simulink model "ALL_JP360_DBW_V6_5_1103"  (R2022a)
settings: Solver=FixedStepAuto  StartTime=0.0  StopTime=inf  FixedStep=0.01  RelTol=1e-3  EnableMultiTasking=on
model workspace (MAT data in the model file):
  g = 9.8
undefined symbols (not defined in the file or in its folder): canChannel, delta_v_p, IPM_Line_C0, IPM_Line_C1, IPM_Line_C2, IPM_Line_C3, M, M_p, MRR_ObjDistX, MRR_ObjDistY, MRR_ObjFusionCamID, MRR_ObjFusionSig, MRR_ObjID, MRR_ObjRelVelX, MRR_ObjRelVelY, MRR_ObjType, MRR_ObjUpdFlg, none, obj_vaild, untracktime, V, videoinput
libraries: canfdmsglib x230, canfdlib x76, slpidlib x24, simulink x18, dspstat3 x14, ctrlSharedLib x1, simulink_extras x1, imaqlib x1, realtime_pacer_lib x1, dspvision x1, visionsinks x1
(part 40 of 55)

== system ALL_JP360_DBW_V6_5_1103/MsgFromCAN/Subsystem/Subsystem3 ==
  VR_ADCU_MRR_ObjHeader_0x680FromOutData : Inport
  Bus Selector : BusSelector  OutputSignals=MRR_ObjDistX_07,MRR_ObjDistY_07,MRR_ObjExistProb_07,MRR_ObjFusionCamID_07,MRR_ObjFusionSig_07,MRR_ObjID_07,MRR_ObjMovingSts_07,MRR_ObjObstacleProb_07,MRR_ObjRelAccelX_07,MRR_ObjRelAccelY_07,MRR_ObjRelVelX_07,MRR_ObjRelVelY_07,MRR_ObjType_07,MRR_ObjUpdFlg_07
  Bus Selector1 : BusSelector  OutputSignals=MRR_ObjDistX_08,MRR_ObjDistY_08,MRR_ObjExistProb_08,MRR_ObjFusionCamID_08,MRR_ObjFusionSig_08,MRR_ObjID_08,MRR_ObjMovingSts_08,MRR_ObjObstacleProb_08,MRR_ObjRelAccelX_08,MRR_ObjRelAccelY_08,MRR_ObjRelVelX_08,MRR_ObjRelVelY_08,MRR_ObjType_08,MRR_ObjUpdFlg_08
  Data Type Conversion{,1..27} (28 alike) : DataTypeConversion  OutDataTypeStr=single  SaturateOnIntegerOverflow=off  RndMeth=Floor
  Mux : Mux  Inputs=14
  Mux1 : Mux  Inputs=14
  Out1 : Outport
  Out2 : Outport  Port=2
  wires:
  Data Type Conversion5/1 -> Mux/6
  Data Type Conversion3/1 -> Mux/4
  Data Type Conversion17/1 -> Mux1/3
  Data Type Conversion19/1 -> Mux1/5
  Data Type Conversion26/1 -> Mux1/12
  Data Type Conversion24/1 -> Mux1/10
  Data Type Conversion22/1 -> Mux1/8
  Data Type Conversion20/1 -> Mux1/6
  Data Type Conversion4/1 -> Mux/5
  Data Type Conversion2/1 -> Mux/3
  Data Type Conversion16/1 -> Mux1/2
  Data Type Conversion18/1 -> Mux1/4
  Data Type Conversion27/1 -> Mux1/13
  Data Type Conversion25/1 -> Mux1/11
  Data Type Conversion23/1 -> Mux1/9
  Data Type Conversion21/1 -> Mux1/7
  Data Type Conversion13/1 -> Mux/14
  Data Type Conversion11/1 -> Mux/12
  Data Type Conversion1/1 -> Mux/2
  Data Type Conversion15/1 -> Mux1/1
  Bus Selector1/11 -> Data Type Conversion25/1  "<MRR_ObjRelVelX_08>"
  Bus Selector1/13 -> Data Type Conversion27/1  "<MRR_ObjType_08>"
  Bus Selector1/10 -> Data Type Conversion24/1  "<MRR_ObjRelAccelY_08>"
  Bus Selector1/12 -> Data Type Conversion26/1  "<MRR_ObjRelVelY_08>"
  Bus Selector/3 -> Data Type Conversion2/1  "<MRR_ObjExistProb_07>"
  Bus Selector1/5 -> Data Type Conversion19/1  "<MRR_ObjFusionSig_08>"
  Bus Selector1/7 -> Data Type Conversion21/1  "<MRR_ObjMovingSts_08>"
  Bus Selector1/9 -> Data Type Conversion23/1  "<MRR_ObjRelAccelX_08>"
  Bus Selector/14 -> Data Type Conversion13/1  "<MRR_ObjUpdFlg_07>"
  Bus Selector1/4 -> Data Type Conversion18/1  "<MRR_ObjFusionCamID_08>"
  Bus Selector1/6 -> Data Type Conversion20/1  "<MRR_ObjID_08>"
  Bus Selector1/8 -> Data Type Conversion22/1  "<MRR_ObjObstacleProb_08>"
  Bus Selector1/3 -> Data Type Conversion17/1  "<MRR_ObjExistProb_08>"
  Bus Selector1/2 -> Data Type Conversion16/1  "<MRR_ObjDistY_08>"
  Bus Selector1/1 -> Data Type Conversion15/1  "<MRR_ObjDistX_08>"
  Data Type Conversion12/1 -> Mux/13
  Data Type Conversion10/1 -> Mux/11
  Data Type Conversion/1 -> Mux/1
  Data Type Conversion8/1 -> Mux/9
  Data Type Conversion6/1 -> Mux/7
  Data Type Conversion9/1 -> Mux/10
  Data Type Conversion7/1 -> Mux/8
  Bus Selector/1 -> Data Type Conversion/1  "<MRR_ObjDistX_07>"
  Mux/1 -> Out1/1
  Bus Selector/2 -> Data Type Conversion1/1  "<MRR_ObjDistY_07>"
  Bus Selector/4 -> Data Type Conversion3/1  "<MRR_ObjFusionCamID_07>"
  Bus Selector/5 -> Data Type Conversion4/1  "<MRR_ObjFusionSig_07>"
  Bus Selector/12 -> Data Type Conversion11/1  "<MRR_ObjRelVelY_07>"
  Bus Selector/10 -> Data Type Conversion9/1  "<MRR_ObjRelAccelY_07>"
  Bus Selector/8 -> Data Type Conversion7/1  "<MRR_ObjObstacleProb_07>"
  Bus Selector/6 -> Data Type Conversion5/1  "<MRR_ObjID_07>"
  Bus Selector/13 -> Data Type Conversion12/1  "<MRR_ObjType_07>"
  Bus Selector/11 -> Data Type Conversion10/1  "<MRR_ObjRelVelX_07>"
  Bus Selector/9 -> Data Type Conversion8/1  "<MRR_ObjRelAccelX_07>"
  Bus Selector/7 -> Data Type Conversion6/1  "<MRR_ObjMovingSts_07>"
  Mux1/1 -> Out2/1
  VR_ADCU_MRR_ObjHeader_0x680FromOutData/1 -> Bus Selector1/1, Bus Selector/1

== system ALL_JP360_DBW_V6_5_1103/MsgFromCAN/Subsystem/Subsystem4 ==
  VR_ADCU_MRR_ObjHeader_0x680FromOutData : Inport
  Bus Selector : BusSelector  OutputSignals=MRR_ObjDistX_09,MRR_ObjDistY_09,MRR_ObjExistProb_09,MRR_ObjFusionCamID_09,MRR_ObjFusionSig_09,MRR_ObjID_09,MRR_ObjMovingSts_09,MRR_ObjObstacleProb_09,MRR_ObjRelAccelX_09,MRR_ObjRelAccelY_09,MRR_ObjRelVelX_09,MRR_ObjRelVelY_09,MRR_ObjType_09,MRR_ObjUpdFlg_09
  Bus Selector1 : BusSelector  OutputSignals=MRR_ObjDistX_10,MRR_ObjDistY_10,MRR_ObjExistProb_10,MRR_ObjFusionCamID_10,MRR_ObjFusionSig_10,MRR_ObjID_10,MRR_ObjMovingSts_10,MRR_ObjObstacleProb_10,MRR_ObjRelAccelX_10,MRR_ObjRelAccelY_10,MRR_ObjRelVelX_10,MRR_ObjRelVelY_10,MRR_ObjType_10,MRR_ObjUpdFlg_10
  Data Type Conversion{,1..27} (28 alike) : DataTypeConversion  OutDataTypeStr=single  SaturateOnIntegerOverflow=off  RndMeth=Floor
  Mux : Mux  Inputs=14
  Mux1 : Mux  Inputs=14
  Out1 : Outport
  Out2 : Outport  Port=2
  wires:
  Mux/1 -> Out1/1
  Mux1/1 -> Out2/1
  VR_ADCU_MRR_ObjHeader_0x680FromOutData/1 -> Bus Selector/1, Bus Selector1/1
  Bus Selector/12 -> Data Type Conversion11/1  "<MRR_ObjRelVelY_09>"
  Bus Selector/11 -> Data Type Conversion10/1  "<MRR_ObjRelVelX_09>"
  Bus Selector/13 -> Data Type Conversion12/1  "<MRR_ObjType_09>"
  Bus Selector/10 -> Data Type Conversion9/1  "<MRR_ObjRelAccelY_09>"
  Bus Selector/14 -> Data Type Conversion13/1  "<MRR_ObjUpdFlg_09>"
  Bus Selector/9 -> Data Type Conversion8/1  "<MRR_ObjRelAccelX_09>"
  Bus Selector/8 -> Data Type Conversion7/1  "<MRR_ObjObstacleProb_09>"
  Bus Selector/7 -> Data Type Conversion6/1  "<MRR_ObjMovingSts_09>"
  Bus Selector/6 -> Data Type Conversion5/1  "<MRR_ObjID_09>"
  Bus Selector/5 -> Data Type Conversion4/1  "<MRR_ObjFusionSig_09>"
  Bus Selector/4 -> Data Type Conversion3/1  "<MRR_ObjFusionCamID_09>"
  Bus Selector/3 -> Data Type Conversion2/1  "<MRR_ObjExistProb_09>"
  Bus Selector/2 -> Data Type Conversion1/1  "<MRR_ObjDistY_09>"
  Bus Selector/1 -> Data Type Conversion/1  "<MRR_ObjDistX_09>"
  Data Type Conversion11/1 -> Mux/12
  Data Type Conversion10/1 -> Mux/11
  Data Type Conversion12/1 -> Mux/13
  Data Type Conversion9/1 -> Mux/10
  Data Type Conversion13/1 -> Mux/14
  Data Type Conversion8/1 -> Mux/9
  Data Type Conversion7/1 -> Mux/8
  Data Type Conversion6/1 -> Mux/7
  Data Type Conversion5/1 -> Mux/6
  Data Type Conversion4/1 -> Mux/5
  Data Type Conversion3/1 -> Mux/4
  Data Type Conversion2/1 -> Mux/3
  Data Type Conversion1/1 -> Mux/2
  Data Type Conversion/1 -> Mux/1
  Bus Selector1/1 -> Data Type Conversion14/1  "<MRR_ObjDistX_10>"
  Bus Selector1/2 -> Data Type Conversion15/1  "<MRR_ObjDistY_10>"
  Bus Selector1/3 -> Data Type Conversion16/1  "<MRR_ObjExistProb_10>"
  Bus Selector1/4 -> Data Type Conversion17/1  "<MRR_ObjFusionCamID_10>"
  Bus Selector1/5 -> Data Type Conversion18/1  "<MRR_ObjFusionSig_10>"
  Bus Selector1/6 -> Data Type Conversion19/1  "<MRR_ObjID_10>"
  Bus Selector1/7 -> Data Type Conversion20/1  "<MRR_ObjMovingSts_10>"
  Bus Selector1/8 -> Data Type Conversion21/1  "<MRR_ObjObstacleProb_10>"
  Bus Selector1/9 -> Data Type Conversion22/1  "<MRR_ObjRelAccelX_10>"
  Bus Selector1/10 -> Data Type Conversion23/1  "<MRR_ObjRelAccelY_10>"
  Bus Selector1/11 -> Data Type Conversion24/1  "<MRR_ObjRelVelX_10>"
  Bus Selector1/12 -> Data Type Conversion25/1  "<MRR_ObjRelVelY_10>"
  Bus Selector1/13 -> Data Type Conversion26/1  "<MRR_ObjType_10>"
  Bus Selector1/14 -> Data Type Conversion27/1  "<MRR_ObjUpdFlg_10>"
  Data Type Conversion14/1 -> Mux1/1
  Data Type Conversion15/1 -> Mux1/2
  Data Type Conversion16/1 -> Mux1/3
  Data Type Conversion17/1 -> Mux1/4
  Data Type Conversion18/1 -> Mux1/5
  Data Type Conversion19/1 -> Mux1/6
  Data Type Conversion20/1 -> Mux1/7
  Data Type Conversion21/1 -> Mux1/8
  Data Type Conversion22/1 -> Mux1/9
  Data Type Conversion23/1 -> Mux1/10
  Data Type Conversion24/1 -> Mux1/11
  Data Type Conversion25/1 -> Mux1/12
  Data Type Conversion26/1 -> Mux1/13
  Data Type Conversion27/1 -> Mux1/14

== system ALL_JP360_DBW_V6_5_1103/MsgFromCAN/Subsystem/Subsystem5 ==
  VR_ADCU_MRR_ObjHeader_0x680FromOutData : Inport
  Bus Selector : BusSelector  OutputSignals=MRR_ObjDistX_11,MRR_ObjDistY_11,MRR_ObjExistProb_11,MRR_ObjFusionCamID_11,MRR_ObjFusionSig_11,MRR_ObjID_11,MRR_ObjMovingSts_11,MRR_ObjObstacleProb_11,MRR_ObjRelAccelX_11,MRR_ObjRelAccelY_11,MRR_ObjRelVelX_11,MRR_ObjRelVelY_11,MRR_ObjType_11,MRR_ObjUpdFlg_11
  Bus Selector1 : BusSelector  OutputSignals=MRR_ObjDistX_12,MRR_ObjDistY_12,MRR_ObjExistProb_12,MRR_ObjFusionCamID_12,MRR_ObjFusionSig_12,MRR_ObjID_12,MRR_ObjMovingSts_12,MRR_ObjObstacleProb_12,MRR_ObjRelAccelX_12,MRR_ObjRelAccelY_12,MRR_ObjRelVelX_12,MRR_ObjRelVelY_12,MRR_ObjType_12,MRR_ObjUpdFlg_12
  Data Type Conversion{,1..27} (28 alike) : DataTypeConversion  OutDataTypeStr=single  SaturateOnIntegerOverflow=off  RndMeth=Floor
  Mux : Mux  Inputs=14
  Mux1 : Mux  Inputs=14
  Out1 : Outport
  Out2 : Outport  Port=2
  wires:
  VR_ADCU_MRR_ObjHeader_0x680FromOutData/1 -> Bus Selector1/1, Bus Selector/1
  Mux1/1 -> Out2/1
  Mux/1 -> Out1/1
  Bus Selector/10 -> Data Type Conversion9/1  "<MRR_ObjRelAccelY_11>"
  Bus Selector/11 -> Data Type Conversion10/1  "<MRR_ObjRelVelX_11>"
  Bus Selector/9 -> Data Type Conversion8/1  "<MRR_ObjRelAccelX_11>"
  Bus Selector/12 -> Data Type Conversion11/1  "<MRR_ObjRelVelY_11>"
  Bus Selector/8 -> Data Type Conversion7/1  "<MRR_ObjObstacleProb_11>"
  Bus Selector/13 -> Data Type Conversion12/1  "<MRR_ObjType_11>"
  Bus Selector/7 -> Data Type Conversion6/1  "<MRR_ObjMovingSts_11>"
  Bus Selector/14 -> Data Type Conversion13/1  "<MRR_ObjUpdFlg_11>"
  Bus Selector/6 -> Data Type Conversion5/1  "<MRR_ObjID_11>"
  Bus Selector/5 -> Data Type Conversion4/1  "<MRR_ObjFusionSig_11>"
  Bus Selector/4 -> Data Type Conversion3/1  "<MRR_ObjFusionCamID_11>"
  Bus Selector/3 -> Data Type Conversion2/1  "<MRR_ObjExistProb_11>"
  Bus Selector/2 -> Data Type Conversion1/1  "<MRR_ObjDistY_11>"
  Bus Selector/1 -> Data Type Conversion/1  "<MRR_ObjDistX_11>"
  Data Type Conversion9/1 -> Mux/10
  Data Type Conversion10/1 -> Mux/11
  Data Type Conversion8/1 -> Mux/9
  Data Type Conversion11/1 -> Mux/12
  Data Type Conversion7/1 -> Mux/8
  Data Type Conversion12/1 -> Mux/13
  Data Type Conversion6/1 -> Mux/7
  Data Type Conversion13/1 -> Mux/14
  Data Type Conversion5/1 -> Mux/6
  Data Type Conversion4/1 -> Mux/5
  Data Type Conversion3/1 -> Mux/4
  Data Type Conversion2/1 -> Mux/3
  Data Type Conversion1/1 -> Mux/2
  Data Type Conversion/1 -> Mux/1
  Bus Selector1/1 -> Data Type Conversion14/1  "<MRR_ObjDistX_12>"
  Bus Selector1/2 -> Data Type Conversion15/1  "<MRR_ObjDistY_12>"
  Bus Selector1/3 -> Data Type Conversion16/1  "<MRR_ObjExistProb_12>"
  Bus Selector1/4 -> Data Type Conversion17/1  "<MRR_ObjFusionCamID_12>"
  Bus Selector1/5 -> Data Type Conversion18/1  "<MRR_ObjFusionSig_12>"
  Bus Selector1/6 -> Data Type Conversion19/1  "<MRR_ObjID_12>"
  Bus Selector1/7 -> Data Type Conversion20/1  "<MRR_ObjMovingSts_12>"
  Bus Selector1/8 -> Data Type Conversion21/1  "<MRR_ObjObstacleProb_12>"
  Bus Selector1/9 -> Data Type Conversion22/1  "<MRR_ObjRelAccelX_12>"
  Bus Selector1/10 -> Data Type Conversion23/1  "<MRR_ObjRelAccelY_12>"
  Bus Selector1/11 -> Data Type Conversion24/1  "<MRR_ObjRelVelX_12>"
  Bus Selector1/12 -> Data Type Conversion25/1  "<MRR_ObjRelVelY_12>"
  Bus Selector1/13 -> Data Type Conversion26/1  "<MRR_ObjType_12>"
  Bus Selector1/14 -> Data Type Conversion27/1  "<MRR_ObjUpdFlg_12>"
  Data Type Conversion14/1 -> Mux1/1
  Data Type Conversion15/1 -> Mux1/2
  Data Type Conversion16/1 -> Mux1/3
  Data Type Conversion17/1 -> Mux1/4
  Data Type Conversion18/1 -> Mux1/5
  Data Type Conversion19/1 -> Mux1/6
  Data Type Conversion20/1 -> Mux1/7
  Data Type Conversion21/1 -> Mux1/8
  Data Type Conversion22/1 -> Mux1/9
  Data Type Conversion23/1 -> Mux1/10
  Data Type Conversion24/1 -> Mux1/11
  Data Type Conversion25/1 -> Mux1/12
  Data Type Conversion26/1 -> Mux1/13
  Data Type Conversion27/1 -> Mux1/14

== system ALL_JP360_DBW_V6_5_1103/MsgFromCAN/Subsystem/Subsystem6 ==
  VR_ADCU_MRR_ObjHeader_0x680FromOutData : Inport
  Bus Selector : BusSelector  OutputSignals=MRR_ObjDistX_13,MRR_ObjDistY_13,MRR_ObjExistProb_13,MRR_ObjFusionCamID_13,MRR_ObjFusionSig_13,MRR_ObjID_13,MRR_ObjMovingSts_13,MRR_ObjObstacleProb_13,MRR_ObjRelAccelX_13,MRR_ObjRelAccelY_13,MRR_ObjRelVelX_13,MRR_ObjRelVelY_13,MRR_ObjType_13,MRR_ObjUpdFlg_13
  Bus Selector1 : BusSelector  OutputSignals=MRR_ObjDistX_14,MRR_ObjDistY_14,MRR_ObjExistProb_14,MRR_ObjFusionCamID_14,MRR_ObjFusionSig_14,MRR_ObjID_14,MRR_ObjMovingSts_14,MRR_ObjObstacleProb_14,MRR_ObjRelAccelX_14,MRR_ObjRelAccelY_14,MRR_ObjRelVelX_14,MRR_ObjRelVelY_14,MRR_ObjType_14,MRR_ObjUpdFlg_14
  Data Type Conversion{,1..27} (28 alike) : DataTypeConversion  OutDataTypeStr=single  SaturateOnIntegerOverflow=off  RndMeth=Floor
  Mux : Mux  Inputs=14
  Mux1 : Mux  Inputs=14
  Out1 : Outport
  Out2 : Outport  Port=2
  wires:
  Bus Selector/13 -> Data Type Conversion12/1  "<MRR_ObjType_13>"
  Bus Selector/1 -> Data Type Conversion/1  "<MRR_ObjDistX_13>"
  Data Type Conversion4/1 -> Mux/5
  Bus Selector1/5 -> Data Type Conversion18/1  "<MRR_ObjFusionSig_14>"
  Bus Selector1/7 -> Data Type Conversion20/1  "<MRR_ObjMovingSts_14>"
  Data Type Conversion27/1 -> Mux1/14
  Data Type Conversion25/1 -> Mux1/12
  Data Type Conversion23/1 -> Mux1/10
  Bus Selector/14 -> Data Type Conversion13/1  "<MRR_ObjUpdFlg_13>"
  Bus Selector/12 -> Data Type Conversion11/1  "<MRR_ObjRelVelY_13>"
  Data Type Conversion5/1 -> Mux/6
  Data Type Conversion3/1 -> Mux/4
  Bus Selector1/4 -> Data Type Conversion17/1  "<MRR_ObjFusionCamID_14>"
  Bus Selector1/6 -> Data Type Conversion19/1  "<MRR_ObjID_14>"
  Data Type Conversion26/1 -> Mux1/13
  Data Type Conversion24/1 -> Mux1/11
  Bus Selector1/2 -> Data Type Conversion15/1  "<MRR_ObjDistY_14>"
  Data Type Conversion17/1 -> Mux1/4
  Data Type Conversion19/1 -> Mux1/6
  Data Type Conversion22/1 -> Mux1/9
  Data Type Conversion20/1 -> Mux1/7
  Bus Selector/2 -> Data Type Conversion1/1  "<MRR_ObjDistY_13>"
  Data Type Conversion2/1 -> Mux/3
  Data Type Conversion16/1 -> Mux1/3
  Data Type Conversion18/1 -> Mux1/5
  Data Type Conversion21/1 -> Mux1/8
  Data Type Conversion13/1 -> Mux/14
  Data Type Conversion11/1 -> Mux/12
  Data Type Conversion1/1 -> Mux/2
  Data Type Conversion15/1 -> Mux1/2
  Data Type Conversion12/1 -> Mux/13
  Data Type Conversion10/1 -> Mux/11
  Data Type Conversion/1 -> Mux/1
  Data Type Conversion14/1 -> Mux1/1
  Data Type Conversion8/1 -> Mux/9
  Data Type Conversion6/1 -> Mux/7
  Bus Selector1/8 -> Data Type Conversion21/1  "<MRR_ObjObstacleProb_14>"
  Bus Selector1/10 -> Data Type Conversion23/1  "<MRR_ObjRelAccelY_14>"
  Bus Selector1/12 -> Data Type Conversion25/1  "<MRR_ObjRelVelY_14>"
  Bus Selector1/14 -> Data Type Conversion27/1  "<MRR_ObjUpdFlg_14>"
  Data Type Conversion9/1 -> Mux/10
  Data Type Conversion7/1 -> Mux/8
  Bus Selector1/9 -> Data Type Conversion22/1  "<MRR_ObjRelAccelX_14>"
  Bus Selector1/11 -> Data Type Conversion24/1  "<MRR_ObjRelVelX_14>"
  Bus Selector1/13 -> Data Type Conversion26/1  "<MRR_ObjType_14>"
  Bus Selector1/3 -> Data Type Conversion16/1  "<MRR_ObjExistProb_14>"
  Bus Selector1/1 -> Data Type Conversion14/1  "<MRR_ObjDistX_14>"
  Bus Selector/3 -> Data Type Conversion2/1  "<MRR_ObjExistProb_13>"
  Bus Selector/10 -> Data Type Conversion9/1  "<MRR_ObjRelAccelY_13>"
  Bus Selector/8 -> Data Type Conversion7/1  "<MRR_ObjObstacleProb_13>"
  Bus Selector/6 -> Data Type Conversion5/1  "<MRR_ObjID_13>"
  Bus Selector/4 -> Data Type Conversion3/1  "<MRR_ObjFusionCamID_13>"
  Bus Selector/11 -> Data Type Conversion10/1  "<MRR_ObjRelVelX_13>"
  Bus Selector/9 -> Data Type Conversion8/1  "<MRR_ObjRelAccelX_13>"
  Bus Selector/7 -> Data Type Conversion6/1  "<MRR_ObjMovingSts_13>"
  Bus Selector/5 -> Data Type Conversion4/1  "<MRR_ObjFusionSig_13>"
  Mux/1 -> Out1/1
  Mux1/1 -> Out2/1
  VR_ADCU_MRR_ObjHeader_0x680FromOutData/1 -> Bus Selector/1, Bus Selector1/1

== system ALL_JP360_DBW_V6_5_1103/MsgFromCAN/Subsystem/Subsystem7 ==
  VR_ADCU_MRR_ObjHeader_0x680FromOutData : Inport
  Bus Selector : BusSelector  OutputSignals=MRR_ObjDistX_15,MRR_ObjDistY_15,MRR_ObjExistProb_15,MRR_ObjFusionCamID_15,MRR_ObjFusionSig_15,MRR_ObjID_15,MRR_ObjMovingSts_15,MRR_ObjObstacleProb_15,MRR_ObjRelAccelX_15,MRR_ObjRelAccelY_15,MRR_ObjRelVelX_15,MRR_ObjRelVelY_15,MRR_ObjType_15,MRR_ObjUpdFlg_15
  Bus Selector1 : BusSelector  OutputSignals=MRR_ObjDistX_16,MRR_ObjDistY_16,MRR_ObjExistProb_16,MRR_ObjFusionCamID_16,MRR_ObjFusionSig_16,MRR_ObjID_16,MRR_ObjMovingSts_16,MRR_ObjObstacleProb_16,MRR_ObjRelAccelX_16,MRR_ObjRelAccelY_16,MRR_ObjRelVelX_16,MRR_ObjRelVelY_16,MRR_ObjType_16,MRR_ObjUpdFlg_16
  Data Type Conversion{,1..27} (28 alike) : DataTypeConversion  OutDataTypeStr=single  SaturateOnIntegerOverflow=off  RndMeth=Floor
  Mux : Mux  Inputs=14
  Mux1 : Mux  Inputs=14
  Out1 : Outport
  Out2 : Outport  Port=2
  wires:
  Bus Selector1/12 -> Data Type Conversion27/1  "<MRR_ObjRelVelY_16>"
  Bus Selector1/10 -> Data Type Conversion25/1  "<MRR_ObjRelAccelY_16>"
  Bus Selector1/11 -> Data Type Conversion26/1  "<MRR_ObjRelVelX_16>"
  Bus Selector1/9 -> Data Type Conversion24/1  "<MRR_ObjRelAccelX_16>"
  Bus Selector1/7 -> Data Type Conversion22/1  "<MRR_ObjMovingSts_16>"
  Bus Selector1/5 -> Data Type Conversion20/1  "<MRR_ObjFusionSig_16>"
  Bus Selector/14 -> Data Type Conversion13/1  "<MRR_ObjUpdFlg_15>"
  Bus Selector1/4 -> Data Type Conversion19/1  "<MRR_ObjFusionCamID_16>"
  Bus Selector1/8 -> Data Type Conversion23/1  "<MRR_ObjObstacleProb_16>"
  Bus Selector1/6 -> Data Type Conversion21/1  "<MRR_ObjID_16>"
  Bus Selector1/3 -> Data Type Conversion18/1  "<MRR_ObjExistProb_16>"
  Mux1/1 -> Out2/1
  Bus Selector/1 -> Data Type Conversion/1  "<MRR_ObjDistX_15>"
  Bus Selector1/2 -> Data Type Conversion17/1  "<MRR_ObjDistY_16>"
  VR_ADCU_MRR_ObjHeader_0x680FromOutData/1 -> Bus Selector/1, Bus Selector1/1
  Bus Selector1/1 -> Data Type Conversion16/1  "<MRR_ObjDistX_16>"
  Data Type Conversion8/1 -> Mux/9
  Data Type Conversion6/1 -> Mux/7
  Data Type Conversion4/1 -> Mux/5
  Data Type Conversion27/1 -> Mux1/12
  Data Type Conversion7/1 -> Mux/8
  Data Type Conversion5/1 -> Mux/6
  Data Type Conversion3/1 -> Mux/4
  Data Type Conversion26/1 -> Mux1/11
  Data Type Conversion2/1 -> Mux/3
  Data Type Conversion21/1 -> Mux1/6
  Data Type Conversion23/1 -> Mux1/8
  Data Type Conversion25/1 -> Mux1/10
  Bus Selector/2 -> Data Type Conversion1/1  "<MRR_ObjDistY_15>"
  Data Type Conversion19/1 -> Mux1/4
  Data Type Conversion20/1 -> Mux1/5
  Data Type Conversion22/1 -> Mux1/7
  Data Type Conversion24/1 -> Mux1/9
  Data Type Conversion12/1 -> Mux/13
  Data Type Conversion16/1 -> Mux1/1
  Data Type Conversion18/1 -> Mux1/3
  Data Type Conversion13/1 -> Mux/14
  Data Type Conversion11/1 -> Mux/12
  Data Type Conversion17/1 -> Mux1/2
  Data Type Conversion10/1 -> Mux/11
  Data Type Conversion/1 -> Mux/1
  Data Type Conversion1/1 -> Mux/2
  Mux/1 -> Out1/1
  Data Type Conversion9/1 -> Mux/10
  Bus Selector/3 -> Data Type Conversion2/1  "<MRR_ObjExistProb_15>"
  Bus Selector/4 -> Data Type Conversion3/1  "<MRR_ObjFusionCamID_15>"
  Bus Selector/5 -> Data Type Conversion4/1  "<MRR_ObjFusionSig_15>"
  Bus Selector/12 -> Data Type Conversion11/1  "<MRR_ObjRelVelY_15>"
  Bus Selector/10 -> Data Type Conversion9/1  "<MRR_ObjRelAccelY_15>"
  Bus Selector/8 -> Data Type Conversion7/1  "<MRR_ObjObstacleProb_15>"
  Bus Selector/6 -> Data Type Conversion5/1  "<MRR_ObjID_15>"
  Bus Selector/13 -> Data Type Conversion12/1  "<MRR_ObjType_15>"
  Bus Selector/11 -> Data Type Conversion10/1  "<MRR_ObjRelVelX_15>"
  Bus Selector/9 -> Data Type Conversion8/1  "<MRR_ObjRelAccelX_15>"
  Bus Selector/7 -> Data Type Conversion6/1  "<MRR_ObjMovingSts_15>"

== system ALL_JP360_DBW_V6_5_1103/MsgFromCAN/Subsystem/Subsystem8 ==
  VR_ADCU_MRR_ObjHeader_0x680FromOutData : Inport
  Bus Selector : BusSelector  OutputSignals=MRR_ObjDistX_17,MRR_ObjDistY_17,MRR_ObjExistProb_17,MRR_ObjFusionCamID_17,MRR_ObjFusionSig_17,MRR_ObjID_17,MRR_ObjMovingSts_17,MRR_ObjObstacleProb_17,MRR_ObjRelAccelX_17,MRR_ObjRelAccelY_17,MRR_ObjRelVelX_17,MRR_ObjRelVelY_17,MRR_ObjType_17,MRR_ObjUpdFlg_17
  Bus Selector1 : BusSelector  OutputSignals=MRR_ObjDistX_18,MRR_ObjDistY_18,MRR_ObjExistProb_18,MRR_ObjFusionCamID_18,MRR_ObjFusionSig_18,MRR_ObjID_18,MRR_ObjMovingSts_18,MRR_ObjObstacleProb_18,MRR_ObjRelAccelX_18,MRR_ObjRelAccelY_18,MRR_ObjRelVelX_18,MRR_ObjRelVelY_18,MRR_ObjType_18,MRR_ObjUpdFlg_18
  Data Type Conversion{,1..27} (28 alike) : DataTypeConversion  OutDataTypeStr=single  SaturateOnIntegerOverflow=off  RndMeth=Floor
  Mux : Mux  Inputs=14
  Mux1 : Mux  Inputs=14
  Out1 : Outport
  Out2 : Outport  Port=2
  wires:
  Data Type Conversion4/1 -> Mux/5
  Data Type Conversion6/1 -> Mux/7
  Data Type Conversion27/1 -> Mux1/14
  Data Type Conversion25/1 -> Mux1/12
  Data Type Conversion3/1 -> Mux/4
  Data Type Conversion5/1 -> Mux/6
  Data Type Conversion7/1 -> Mux/8
  Data Type Conversion26/1 -> Mux1/13
  Data Type Conversion19/1 -> Mux1/6
  Data Type Conversion24/1 -> Mux1/11
  Data Type Conversion22/1 -> Mux1/9
  Data Type Conversion20/1 -> Mux1/7
  Data Type Conversion2/1 -> Mux/3
  Data Type Conversion18/1 -> Mux1/5
  Data Type Conversion23/1 -> Mux1/10
  Data Type Conversion21/1 -> Mux1/8
  Data Type Conversion11/1 -> Mux/12
  Data Type Conversion13/1 -> Mux/14
  Data Type Conversion15/1 -> Mux1/2
  Data Type Conversion17/1 -> Mux1/4
  Data Type Conversion10/1 -> Mux/11
  Data Type Conversion12/1 -> Mux/13
  Data Type Conversion14/1 -> Mux1/1
  Data Type Conversion16/1 -> Mux1/3
  Bus Selector1/12 -> Data Type Conversion25/1  "<MRR_ObjRelVelY_18>"
  Bus Selector1/14 -> Data Type Conversion27/1  "<MRR_ObjUpdFlg_18>"
  Bus Selector1/13 -> Data Type Conversion26/1  "<MRR_ObjType_18>"
  Mux1/1 -> Out2/1
  Bus Selector1/5 -> Data Type Conversion18/1  "<MRR_ObjFusionSig_18>"
  Bus Selector1/7 -> Data Type Conversion20/1  "<MRR_ObjMovingSts_18>"
  Bus Selector1/9 -> Data Type Conversion22/1  "<MRR_ObjRelAccelX_18>"
  Bus Selector1/11 -> Data Type Conversion24/1  "<MRR_ObjRelVelX_18>"
  Bus Selector1/4 -> Data Type Conversion17/1  "<MRR_ObjFusionCamID_18>"
  Bus Selector1/6 -> Data Type Conversion19/1  "<MRR_ObjID_18>"
  Bus Selector1/8 -> Data Type Conversion21/1  "<MRR_ObjObstacleProb_18>"
  Bus Selector1/10 -> Data Type Conversion23/1  "<MRR_ObjRelAccelY_18>"
  Bus Selector1/3 -> Data Type Conversion16/1  "<MRR_ObjExistProb_18>"
  Data Type Conversion1/1 -> Mux/2
  Bus Selector1/2 -> Data Type Conversion15/1  "<MRR_ObjDistY_18>"
  Data Type Conversion8/1 -> Mux/9
  Bus Selector1/1 -> Data Type Conversion14/1  "<MRR_ObjDistX_18>"
  Data Type Conversion9/1 -> Mux/10
  Data Type Conversion/1 -> Mux/1
  Bus Selector/8 -> Data Type Conversion7/1  "<MRR_ObjObstacleProb_17>"
  Bus Selector/10 -> Data Type Conversion9/1  "<MRR_ObjRelAccelY_17>"
  Bus Selector/12 -> Data Type Conversion11/1  "<MRR_ObjRelVelY_17>"
  Bus Selector/14 -> Data Type Conversion13/1  "<MRR_ObjUpdFlg_17>"
  Bus Selector/3 -> Data Type Conversion2/1  "<MRR_ObjExistProb_17>"
  Bus Selector/9 -> Data Type Conversion8/1  "<MRR_ObjRelAccelX_17>"
  Bus Selector/11 -> Data Type Conversion10/1  "<MRR_ObjRelVelX_17>"
  Bus Selector/13 -> Data Type Conversion12/1  "<MRR_ObjType_17>"
  Bus Selector/5 -> Data Type Conversion4/1  "<MRR_ObjFusionSig_17>"
  Bus Selector/7 -> Data Type Conversion6/1  "<MRR_ObjMovingSts_17>"
  Bus Selector/4 -> Data Type Conversion3/1  "<MRR_ObjFusionCamID_17>"
  Bus Selector/6 -> Data Type Conversion5/1  "<MRR_ObjID_17>"
  Bus Selector/1 -> Data Type Conversion/1  "<MRR_ObjDistX_17>"
  Bus Selector/2 -> Data Type Conversion1/1  "<MRR_ObjDistY_17>"
  Mux/1 -> Out1/1
  VR_ADCU_MRR_ObjHeader_0x680FromOutData/1 -> Bus Selector/1, Bus Selector1/1

== system ALL_JP360_DBW_V6_5_1103/MsgFromCAN/Subsystem/Subsystem9 ==
  VR_ADCU_MRR_ObjHeader_0x680FromOutData : Inport
  Bus Selector : BusSelector  OutputSignals=MRR_ObjDistX_19,MRR_ObjDistY_19,MRR_ObjExistProb_19,MRR_ObjFusionCamID_19,MRR_ObjFusionSig_19,MRR_ObjID_19,MRR_ObjMovingSts_19,MRR_ObjObstacleProb_19,MRR_ObjRelAccelX_19,MRR_ObjRelAccelY_19,MRR_ObjRelVelX_19,MRR_ObjRelVelY_19,MRR_ObjType_19,MRR_ObjUpdFlg_19
  Bus Selector1 : BusSelector  OutputSignals=MRR_ObjDistX_20,MRR_ObjDistY_20,MRR_ObjExistProb_20,MRR_ObjFusionCamID_20,MRR_ObjFusionSig_20,MRR_ObjID_20,MRR_ObjMovingSts_20,MRR_ObjObstacleProb_20,MRR_ObjRelAccelX_20,MRR_ObjRelAccelY_20,MRR_ObjRelVelX_20,MRR_ObjRelVelY_20,MRR_ObjType_20,MRR_ObjUpdFlg_20
  Data Type Conversion{,1..27} (28 alike) : DataTypeConversion  OutDataTypeStr=single  SaturateOnIntegerOverflow=off  RndMeth=Floor
  Mux : Mux  Inputs=14
  Mux1 : Mux  Inputs=14
  Out1 : Outport
  Out2 : Outport  Port=2
  wires:
  VR_ADCU_MRR_ObjHeader_0x680FromOutData/1 -> Bus Selector1/1, Bus Selector/1
  Mux1/1 -> Out2/1
  Mux/1 -> Out1/1
  Bus Selector/11 -> Data Type Conversion10/1  "<MRR_ObjRelVelX_19>"
  Bus Selector/12 -> Data Type Conversion11/1  "<MRR_ObjRelVelY_19>"
  Bus Selector/10 -> Data Type Conversion9/1  "<MRR_ObjRelAccelY_19>"
  Bus Selector/13 -> Data Type Conversion12/1  "<MRR_ObjType_19>"
  Bus Selector/9 -> Data Type Conversion8/1  "<MRR_ObjRelAccelX_19>"
  Bus Selector/14 -> Data Type Conversion13/1  "<MRR_ObjUpdFlg_19>"
  Bus Selector/8 -> Data Type Conversion7/1  "<MRR_ObjObstacleProb_19>"
  Bus Selector/7 -> Data Type Conversion6/1  "<MRR_ObjMovingSts_19>"
  Bus Selector/6 -> Data Type Conversion5/1  "<MRR_ObjID_19>"
  Bus Selector/5 -> Data Type Conversion4/1  "<MRR_ObjFusionSig_19>"
  Bus Selector/4 -> Data Type Conversion3/1  "<MRR_ObjFusionCamID_19>"
  Bus Selector/3 -> Data Type Conversion2/1  "<MRR_ObjExistProb_19>"
  Bus Selector/2 -> Data Type Conversion1/1  "<MRR_ObjDistY_19>"
  Bus Selector/1 -> Data Type Conversion/1  "<MRR_ObjDistX_19>"
  Data Type Conversion10/1 -> Mux/11
  Data Type Conversion11/1 -> Mux/12
  Data Type Conversion9/1 -> Mux/10
  Data Type Conversion12/1 -> Mux/13
  Data Type Conversion8/1 -> Mux/9
  Data Type Conversion13/1 -> Mux/14
  Data Type Conversion7/1 -> Mux/8
  Data Type Conversion6/1 -> Mux/7
  Data Type Conversion5/1 -> Mux/6
  Data Type Conversion4/1 -> Mux/5
  Data Type Conversion3/1 -> Mux/4
  Data Type Conversion2/1 -> Mux/3
  Data Type Conversion1/1 -> Mux/2
  Data Type Conversion/1 -> Mux/1
  Bus Selector1/1 -> Data Type Conversion14/1  "<MRR_ObjDistX_20>"
  Bus Selector1/2 -> Data Type Conversion15/1  "<MRR_ObjDistY_20>"
  Bus Selector1/3 -> Data Type Conversion16/1  "<MRR_ObjExistProb_20>"
  Bus Selector1/4 -> Data Type Conversion17/1  "<MRR_ObjFusionCamID_20>"
  Bus Selector1/5 -> Data Type Conversion18/1  "<MRR_ObjFusionSig_20>"
  Bus Selector1/6 -> Data Type Conversion19/1  "<MRR_ObjID_20>"
  Bus Selector1/7 -> Data Type Conversion20/1  "<MRR_ObjMovingSts_20>"
  Bus Selector1/8 -> Data Type Conversion21/1  "<MRR_ObjObstacleProb_20>"
  Bus Selector1/9 -> Data Type Conversion22/1  "<MRR_ObjRelAccelX_20>"
  Bus Selector1/10 -> Data Type Conversion23/1  "<MRR_ObjRelAccelY_20>"
  Bus Selector1/11 -> Data Type Conversion24/1  "<MRR_ObjRelVelX_20>"
  Bus Selector1/12 -> Data Type Conversion25/1  "<MRR_ObjRelVelY_20>"
  Bus Selector1/13 -> Data Type Conversion26/1  "<MRR_ObjType_20>"
  Bus Selector1/14 -> Data Type Conversion27/1  "<MRR_ObjUpdFlg_20>"
  Data Type Conversion14/1 -> Mux1/1
  Data Type Conversion15/1 -> Mux1/2
  Data Type Conversion16/1 -> Mux1/3
  Data Type Conversion17/1 -> Mux1/4
  Data Type Conversion18/1 -> Mux1/5
  Data Type Conversion19/1 -> Mux1/6
  Data Type Conversion20/1 -> Mux1/7
  Data Type Conversion21/1 -> Mux1/8
  Data Type Conversion22/1 -> Mux1/9
  Data Type Conversion23/1 -> Mux1/10
  Data Type Conversion24/1 -> Mux1/11
  Data Type Conversion25/1 -> Mux1/12
  Data Type Conversion26/1 -> Mux1/13
  Data Type Conversion27/1 -> Mux1/14

== system ALL_JP360_DBW_V6_5_1103/MsgFromCAN/Subsystem1/Subsystem1 ==
  VR_ADCU_MRR_ObjHeader_0x680FromOutData : Inport
  Bus Selector1 : BusSelector  OutputSignals=IPM_ObjBlockCounter_02,IPM_ObjDistX_02,IPM_ObjDistY_02,IPM_ObjID_02,IPM_ObjRelAccelX_02,IPM_ObjRelAccelY_02,IPM_ObjRelVelX_02,IPM_ObjRelVelY_02,IPM_ObjType_02,IPM_Object_Age_02,IPM_Object_Existence_Probability_02,IPM_Object_Heading_02,IPM_Object_Height_02,IPM_Object_Length_02,IPM_Object_Motion_Status_02,IPM_Object_Width_02
  Data Type Conversion{1..2,4,6,16..27} (16 alike) : DataTypeConversion  OutDataTypeStr=single  SaturateOnIntegerOverflow=off  RndMeth=Floor
  Mux1 : Mux  Inputs=16
  Out2 : Outport
  wires:
  Data Type Conversion6/1 -> Mux1/16
  Data Type Conversion4/1 -> Mux1/15
  Data Type Conversion2/1 -> Mux1/14
  Data Type Conversion1/1 -> Mux1/13
  Bus Selector1/16 -> Data Type Conversion6/1  "<IPM_Object_Width_02>"
  Bus Selector1/15 -> Data Type Conversion4/1  "<IPM_Object_Motion_Status_02>"
  Bus Selector1/14 -> Data Type Conversion2/1  "<IPM_Object_Length_02>"
  Bus Selector1/13 -> Data Type Conversion1/1  "<IPM_Object_Height_02>"
  Data Type Conversion17/1 -> Mux1/2
  Data Type Conversion18/1 -> Mux1/3
  Data Type Conversion16/1 -> Mux1/1
  Data Type Conversion24/1 -> Mux1/9
  Data Type Conversion22/1 -> Mux1/7
  Data Type Conversion20/1 -> Mux1/5
  Data Type Conversion19/1 -> Mux1/4
  Data Type Conversion25/1 -> Mux1/10
  Data Type Conversion23/1 -> Mux1/8
  Data Type Conversion21/1 -> Mux1/6
  Data Type Conversion26/1 -> Mux1/11
  Data Type Conversion27/1 -> Mux1/12
  Bus Selector1/1 -> Data Type Conversion16/1  "<IPM_ObjBlockCounter_02>"
  VR_ADCU_MRR_ObjHeader_0x680FromOutData/1 -> Bus Selector1/1
  Bus Selector1/2 -> Data Type Conversion17/1  "<IPM_ObjDistX_02>"
  Mux1/1 -> Out2/1
  Bus Selector1/3 -> Data Type Conversion18/1  "<IPM_ObjDistY_02>"
  Bus Selector1/6 -> Data Type Conversion21/1  "<IPM_ObjRelAccelY_02>"
  Bus Selector1/8 -> Data Type Conversion23/1  "<IPM_ObjRelVelY_02>"
  Bus Selector1/4 -> Data Type Conversion19/1  "<IPM_ObjID_02>"
  Bus Selector1/5 -> Data Type Conversion20/1  "<IPM_ObjRelAccelX_02>"
  Bus Selector1/7 -> Data Type Conversion22/1  "<IPM_ObjRelVelX_02>"
  Bus Selector1/9 -> Data Type Conversion24/1  "<IPM_ObjType_02>"
  Bus Selector1/11 -> Data Type Conversion26/1  "<IPM_Object_Existence_Probability_02>"
  Bus Selector1/10 -> Data Type Conversion25/1  "<IPM_Object_Age_02>"
  Bus Selector1/12 -> Data Type Conversion27/1  "<IPM_Object_Heading_02>"

== system ALL_JP360_DBW_V6_5_1103/MsgFromCAN/Subsystem1/Subsystem10 ==
  VR_ADCU_MRR_ObjHeader_0x680FromOutData : Inport
  Bus Selector1 : BusSelector  OutputSignals=IPM_ObjBlockCounter_11,IPM_ObjDistX_11,IPM_ObjDistY_11,IPM_ObjID_11,IPM_ObjRelAccelX_11,IPM_ObjRelAccelY_11,IPM_ObjRelVelX_11,IPM_ObjRelVelY_11,IPM_ObjType_11,IPM_Object_Age_11,IPM_Object_Existence_Probability_11,IPM_Object_Heading_11,IPM_Object_Height_11,IPM_Object_Length_11,IPM_Object_Motion_Status_11,IPM_Object_Width_11
  Data Type Conversion{1..2,4,6,16..27} (16 alike) : DataTypeConversion  OutDataTypeStr=single  SaturateOnIntegerOverflow=off  RndMeth=Floor
  Mux1 : Mux  Inputs=16
  Out2 : Outport
  wires:
  Data Type Conversion6/1 -> Mux1/16
  Data Type Conversion4/1 -> Mux1/15
  Data Type Conversion2/1 -> Mux1/14
  Data Type Conversion1/1 -> Mux1/13
  Bus Selector1/16 -> Data Type Conversion6/1  "<IPM_Object_Width_11>"
  Bus Selector1/15 -> Data Type Conversion4/1  "<IPM_Object_Motion_Status_11>"
  Bus Selector1/14 -> Data Type Conversion2/1  "<IPM_Object_Length_11>"
  Bus Selector1/13 -> Data Type Conversion1/1  "<IPM_Object_Height_11>"
  Data Type Conversion17/1 -> Mux1/2
  Data Type Conversion18/1 -> Mux1/3
  Data Type Conversion16/1 -> Mux1/1
  Data Type Conversion24/1 -> Mux1/9
  Data Type Conversion22/1 -> Mux1/7
  Data Type Conversion20/1 -> Mux1/5
  Data Type Conversion19/1 -> Mux1/4
  Data Type Conversion25/1 -> Mux1/10
  Data Type Conversion23/1 -> Mux1/8
  Data Type Conversion21/1 -> Mux1/6
  Data Type Conversion26/1 -> Mux1/11
  Data Type Conversion27/1 -> Mux1/12
  Bus Selector1/1 -> Data Type Conversion16/1  "<IPM_ObjBlockCounter_11>"
  VR_ADCU_MRR_ObjHeader_0x680FromOutData/1 -> Bus Selector1/1
  Bus Selector1/2 -> Data Type Conversion17/1  "<IPM_ObjDistX_11>"
  Mux1/1 -> Out2/1
  Bus Selector1/3 -> Data Type Conversion18/1  "<IPM_ObjDistY_11>"
  Bus Selector1/6 -> Data Type Conversion21/1  "<IPM_ObjRelAccelY_11>"
  Bus Selector1/8 -> Data Type Conversion23/1  "<IPM_ObjRelVelY_11>"
  Bus Selector1/4 -> Data Type Conversion19/1  "<IPM_ObjID_11>"
  Bus Selector1/5 -> Data Type Conversion20/1  "<IPM_ObjRelAccelX_11>"
  Bus Selector1/7 -> Data Type Conversion22/1  "<IPM_ObjRelVelX_11>"
  Bus Selector1/9 -> Data Type Conversion24/1  "<IPM_ObjType_11>"
  Bus Selector1/11 -> Data Type Conversion26/1  "<IPM_Object_Existence_Probability_11>"
  Bus Selector1/10 -> Data Type Conversion25/1  "<IPM_Object_Age_11>"
  Bus Selector1/12 -> Data Type Conversion27/1  "<IPM_Object_Heading_11>"

== system ALL_JP360_DBW_V6_5_1103/MsgFromCAN/Subsystem1/Subsystem11 ==
  VR_ADCU_MRR_ObjHeader_0x680FromOutData : Inport
  Bus Selector1 : BusSelector  OutputSignals=IPM_ObjBlockCounter_12,IPM_ObjDistX_12,IPM_ObjDistY_12,IPM_ObjID_12,IPM_ObjRelAccelX_12,IPM_ObjRelAccelY_12,IPM_ObjRelVelX_12,IPM_ObjRelVelY_12,IPM_ObjType_12,IPM_Object_Age_12,IPM_Object_Existence_Probability_12,IPM_Object_Heading_12,IPM_Object_Height_12,IPM_Object_Length_12,IPM_Object_Motion_Status_12,IPM_Object_Width_12
  Data Type Conversion{1..2,4,6,16..27} (16 alike) : DataTypeConversion  OutDataTypeStr=single  SaturateOnIntegerOverflow=off  RndMeth=Floor
  Mux1 : Mux  Inputs=16
  Out2 : Outport
  wires:
  Bus Selector1/12 -> Data Type Conversion27/1  "<IPM_Object_Heading_12>"
  Bus Selector1/10 -> Data Type Conversion25/1  "<IPM_Object_Age_12>"
  Bus Selector1/11 -> Data Type Conversion26/1  "<IPM_Object_Existence_Probability_12>"
  Bus Selector1/9 -> Data Type Conversion24/1  "<IPM_ObjType_12>"
  Bus Selector1/7 -> Data Type Conversion22/1  "<IPM_ObjRelVelX_12>"
  Bus Selector1/5 -> Data Type Conversion20/1  "<IPM_ObjRelAccelX_12>"
  Bus Selector1/4 -> Data Type Conversion19/1  "<IPM_ObjID_12>"
  Bus Selector1/8 -> Data Type Conversion23/1  "<IPM_ObjRelVelY_12>"
  Bus Selector1/6 -> Data Type Conversion21/1  "<IPM_ObjRelAccelY_12>"
  Bus Selector1/3 -> Data Type Conversion18/1  "<IPM_ObjDistY_12>"
  Mux1/1 -> Out2/1
  Bus Selector1/2 -> Data Type Conversion17/1  "<IPM_ObjDistX_12>"
  VR_ADCU_MRR_ObjHeader_0x680FromOutData/1 -> Bus Selector1/1
  Bus Selector1/1 -> Data Type Conversion16/1  "<IPM_ObjBlockCounter_12>"
  Data Type Conversion27/1 -> Mux1/12
  Data Type Conversion26/1 -> Mux1/11
  Data Type Conversion21/1 -> Mux1/6
  Data Type Conversion23/1 -> Mux1/8
  Data Type Conversion25/1 -> Mux1/10
  Data Type Conversion19/1 -> Mux1/4
  Data Type Conversion20/1 -> Mux1/5
  Data Type Conversion22/1 -> Mux1/7
  Data Type Conversion24/1 -> Mux1/9
  Data Type Conversion16/1 -> Mux1/1
  Data Type Conversion18/1 -> Mux1/3
  Data Type Conversion17/1 -> Mux1/2
  Bus Selector1/13 -> Data Type Conversion1/1  "<IPM_Object_Height_12>"
  Bus Selector1/14 -> Data Type Conversion2/1  "<IPM_Object_Length_12>"
  Bus Selector1/15 -> Data Type Conversion4/1  "<IPM_Object_Motion_Status_12>"
  Bus Selector1/16 -> Data Type Conversion6/1  "<IPM_Object_Width_12>"
  Data Type Conversion1/1 -> Mux1/13
  Data Type Conversion2/1 -> Mux1/14
  Data Type Conversion4/1 -> Mux1/15
  Data Type Conversion6/1 -> Mux1/16

== system ALL_JP360_DBW_V6_5_1103/MsgFromCAN/Subsystem1/Subsystem12 ==
  VR_ADCU_MRR_ObjHeader_0x680FromOutData : Inport
  Bus Selector1 : BusSelector  OutputSignals=IPM_ObjBlockCounter_14,IPM_ObjDistX_14,IPM_ObjDistY_14,IPM_ObjID_14,IPM_ObjRelAccelX_14,IPM_ObjRelAccelY_14,IPM_ObjRelVelX_14,IPM_ObjRelVelY_14,IPM_ObjType_14,IPM_Object_Age_14,IPM_Object_Existence_Probability_14,IPM_Object_Heading_14,IPM_Object_Height_14,IPM_Object_Length_14,IPM_Object_Motion_Status_14,IPM_Object_Width_14
  Data Type Conversion{1..2,4,6,16..27} (16 alike) : DataTypeConversion  OutDataTypeStr=single  SaturateOnIntegerOverflow=off  RndMeth=Floor
  Mux1 : Mux  Inputs=16
  Out2 : Outport
  wires:
  Data Type Conversion6/1 -> Mux1/16
  Data Type Conversion4/1 -> Mux1/15
  Data Type Conversion2/1 -> Mux1/14
  Data Type Conversion1/1 -> Mux1/13
  Bus Selector1/16 -> Data Type Conversion6/1  "<IPM_Object_Width_14>"
  Bus Selector1/15 -> Data Type Conversion4/1  "<IPM_Object_Motion_Status_14>"
  Bus Selector1/14 -> Data Type Conversion2/1  "<IPM_Object_Length_14>"
  Bus Selector1/13 -> Data Type Conversion1/1  "<IPM_Object_Height_14>"
  Data Type Conversion17/1 -> Mux1/2
  Data Type Conversion18/1 -> Mux1/3
  Data Type Conversion16/1 -> Mux1/1
  Data Type Conversion24/1 -> Mux1/9
  Data Type Conversion22/1 -> Mux1/7
  Data Type Conversion20/1 -> Mux1/5
  Data Type Conversion19/1 -> Mux1/4
  Data Type Conversion25/1 -> Mux1/10
  Data Type Conversion23/1 -> Mux1/8
  Data Type Conversion21/1 -> Mux1/6
  Data Type Conversion26/1 -> Mux1/11
  Data Type Conversion27/1 -> Mux1/12
  Bus Selector1/1 -> Data Type Conversion16/1  "<IPM_ObjBlockCounter_14>"
  VR_ADCU_MRR_ObjHeader_0x680FromOutData/1 -> Bus Selector1/1
  Bus Selector1/2 -> Data Type Conversion17/1  "<IPM_ObjDistX_14>"
  Mux1/1 -> Out2/1
  Bus Selector1/3 -> Data Type Conversion18/1  "<IPM_ObjDistY_14>"
  Bus Selector1/6 -> Data Type Conversion21/1  "<IPM_ObjRelAccelY_14>"
  Bus Selector1/8 -> Data Type Conversion23/1  "<IPM_ObjRelVelY_14>"
  Bus Selector1/4 -> Data Type Conversion19/1  "<IPM_ObjID_14>"
  Bus Selector1/5 -> Data Type Conversion20/1  "<IPM_ObjRelAccelX_14>"
  Bus Selector1/7 -> Data Type Conversion22/1  "<IPM_ObjRelVelX_14>"
  Bus Selector1/9 -> Data Type Conversion24/1  "<IPM_ObjType_14>"
  Bus Selector1/11 -> Data Type Conversion26/1  "<IPM_Object_Existence_Probability_14>"
  Bus Selector1/10 -> Data Type Conversion25/1  "<IPM_Object_Age_14>"
  Bus Selector1/12 -> Data Type Conversion27/1  "<IPM_Object_Heading_14>"

== system ALL_JP360_DBW_V6_5_1103/MsgFromCAN/Subsystem1/Subsystem13 ==
  VR_ADCU_MRR_ObjHeader_0x680FromOutData : Inport
  Bus Selector1 : BusSelector  OutputSignals=IPM_ObjBlockCounter_15,IPM_ObjDistX_15,IPM_ObjDistY_15,IPM_ObjID_15,IPM_ObjRelAccelX_15,IPM_ObjRelAccelY_15,IPM_ObjRelVelX_15,IPM_ObjRelVelY_15,IPM_ObjType_15,IPM_Object_Age_15,IPM_Object_Existence_Probability_15,IPM_Object_Heading_15,IPM_Object_Height_15,IPM_Object_Length_15,IPM_Object_Motion_Status_15,IPM_Object_Width_15
  Data Type Conversion{1..2,4,6,16..27} (16 alike) : DataTypeConversion  OutDataTypeStr=single  SaturateOnIntegerOverflow=off  RndMeth=Floor
  Mux1 : Mux  Inputs=16
  Out2 : Outport
  wires:
  Bus Selector1/12 -> Data Type Conversion27/1  "<IPM_Object_Heading_15>"
  Bus Selector1/10 -> Data Type Conversion25/1  "<IPM_Object_Age_15>"
  Bus Selector1/11 -> Data Type Conversion26/1  "<IPM_Object_Existence_Probability_15>"
  Bus Selector1/9 -> Data Type Conversion24/1  "<IPM_ObjType_15>"
  Bus Selector1/7 -> Data Type Conversion22/1  "<IPM_ObjRelVelX_15>"
  Bus Selector1/5 -> Data Type Conversion20/1  "<IPM_ObjRelAccelX_15>"
  Bus Selector1/4 -> Data Type Conversion19/1  "<IPM_ObjID_15>"
  Bus Selector1/8 -> Data Type Conversion23/1  "<IPM_ObjRelVelY_15>"
  Bus Selector1/6 -> Data Type Conversion21/1  "<IPM_ObjRelAccelY_15>"
  Bus Selector1/3 -> Data Type Conversion18/1  "<IPM_ObjDistY_15>"
  Mux1/1 -> Out2/1
  Bus Selector1/2 -> Data Type Conversion17/1  "<IPM_ObjDistX_15>"
  VR_ADCU_MRR_ObjHeader_0x680FromOutData/1 -> Bus Selector1/1
  Bus Selector1/1 -> Data Type Conversion16/1  "<IPM_ObjBlockCounter_15>"
  Data Type Conversion27/1 -> Mux1/12
  Data Type Conversion26/1 -> Mux1/11
  Data Type Conversion21/1 -> Mux1/6
  Data Type Conversion23/1 -> Mux1/8
  Data Type Conversion25/1 -> Mux1/10
  Data Type Conversion19/1 -> Mux1/4
  Data Type Conversion20/1 -> Mux1/5
  Data Type Conversion22/1 -> Mux1/7
  Data Type Conversion24/1 -> Mux1/9
  Data Type Conversion16/1 -> Mux1/1
  Data Type Conversion18/1 -> Mux1/3
  Data Type Conversion17/1 -> Mux1/2
  Bus Selector1/13 -> Data Type Conversion1/1  "<IPM_Object_Height_15>"
  Bus Selector1/14 -> Data Type Conversion2/1  "<IPM_Object_Length_15>"
  Bus Selector1/15 -> Data Type Conversion4/1  "<IPM_Object_Motion_Status_15>"
  Bus Selector1/16 -> Data Type Conversion6/1  "<IPM_Object_Width_15>"
  Data Type Conversion1/1 -> Mux1/13
  Data Type Conversion2/1 -> Mux1/14
  Data Type Conversion4/1 -> Mux1/15
  Data Type Conversion6/1 -> Mux1/16

== system ALL_JP360_DBW_V6_5_1103/MsgFromCAN/Subsystem1/Subsystem14 ==
  VR_ADCU_MRR_ObjHeader_0x680FromOutData : Inport
  Bus Selector1 : BusSelector  OutputSignals=IPM_ObjBlockCounter_13,IPM_ObjDistX_13,IPM_ObjDistY_13,IPM_ObjID_13,IPM_ObjRelAccelX_13,IPM_ObjRelAccelY_13,IPM_ObjRelVelX_13,IPM_ObjRelVelY_13,IPM_ObjType_13,IPM_Object_Age_13,IPM_Object_Existence_Probability_13,IPM_Object_Heading_13,IPM_Object_Height_13,IPM_Object_Length_13,IPM_Object_Motion_Status_13,IPM_Object_Width_13
  Data Type Conversion{1..2,4,6,16..27} (16 alike) : DataTypeConversion  OutDataTypeStr=single  SaturateOnIntegerOverflow=off  RndMeth=Floor
  Mux1 : Mux  Inputs=16
  Out2 : Outport
  wires:
  Bus Selector1/12 -> Data Type Conversion27/1  "<IPM_Object_Heading_13>"
  Bus Selector1/10 -> Data Type Conversion25/1  "<IPM_Object_Age_13>"
  Bus Selector1/11 -> Data Type Conversion26/1  "<IPM_Object_Existence_Probability_13>"
  Bus Selector1/9 -> Data Type Conversion24/1  "<IPM_ObjType_13>"
  Bus Selector1/7 -> Data Type Conversion22/1  "<IPM_ObjRelVelX_13>"
  Bus Selector1/5 -> Data Type Conversion20/1  "<IPM_ObjRelAccelX_13>"
  Bus Selector1/4 -> Data Type Conversion19/1  "<IPM_ObjID_13>"
  Bus Selector1/8 -> Data Type Conversion23/1  "<IPM_ObjRelVelY_13>"
  Bus Selector1/6 -> Data Type Conversion21/1  "<IPM_ObjRelAccelY_13>"
  Bus Selector1/3 -> Data Type Conversion18/1  "<IPM_ObjDistY_13>"
  Mux1/1 -> Out2/1
  Bus Selector1/2 -> Data Type Conversion17/1  "<IPM_ObjDistX_13>"
  VR_ADCU_MRR_ObjHeader_0x680FromOutData/1 -> Bus Selector1/1
  Bus Selector1/1 -> Data Type Conversion16/1  "<IPM_ObjBlockCounter_13>"
  Data Type Conversion27/1 -> Mux1/12
  Data Type Conversion26/1 -> Mux1/11
  Data Type Conversion21/1 -> Mux1/6
  Data Type Conversion23/1 -> Mux1/8
  Data Type Conversion25/1 -> Mux1/10
  Data Type Conversion19/1 -> Mux1/4
  Data Type Conversion20/1 -> Mux1/5
  Data Type Conversion22/1 -> Mux1/7
  Data Type Conversion24/1 -> Mux1/9
  Data Type Conversion16/1 -> Mux1/1
  Data Type Conversion18/1 -> Mux1/3
  Data Type Conversion17/1 -> Mux1/2
  Bus Selector1/13 -> Data Type Conversion1/1  "<IPM_Object_Height_13>"
  Bus Selector1/14 -> Data Type Conversion2/1  "<IPM_Object_Length_13>"
  Bus Selector1/15 -> Data Type Conversion4/1  "<IPM_Object_Motion_Status_13>"
  Bus Selector1/16 -> Data Type Conversion6/1  "<IPM_Object_Width_13>"
  Data Type Conversion1/1 -> Mux1/13
  Data Type Conversion2/1 -> Mux1/14
  Data Type Conversion4/1 -> Mux1/15
  Data Type Conversion6/1 -> Mux1/16

== system ALL_JP360_DBW_V6_5_1103/MsgFromCAN/Subsystem1/Subsystem15 ==
  VR_ADCU_MRR_ObjHeader_0x680FromOutData : Inport
  Bus Selector1 : BusSelector  OutputSignals=IPM_ObjBlockCounter_17,IPM_ObjDistX_17,IPM_ObjDistY_17,IPM_ObjID_17,IPM_ObjRelAccelX_17,IPM_ObjRelAccelY_17,IPM_ObjRelVelX_17,IPM_ObjRelVelY_17,IPM_ObjType_17,IPM_Object_Age_17,IPM_Object_Existence_Probability_17,IPM_Object_Heading_17,IPM_Object_Height_17,IPM_Object_Length_17,IPM_Object_Motion_Status_17,IPM_Object_Width_17
  Data Type Conversion{1..2,4,6,16..27} (16 alike) : DataTypeConversion  OutDataTypeStr=single  SaturateOnIntegerOverflow=off  RndMeth=Floor
  Mux1 : Mux  Inputs=16
  Out2 : Outport
  wires:
  Data Type Conversion6/1 -> Mux1/16
  Data Type Conversion4/1 -> Mux1/15
  Data Type Conversion2/1 -> Mux1/14
  Data Type Conversion1/1 -> Mux1/13
  Bus Selector1/16 -> Data Type Conversion6/1  "<IPM_Object_Width_17>"
  Bus Selector1/15 -> Data Type Conversion4/1  "<IPM_Object_Motion_Status_17>"
  Bus Selector1/14 -> Data Type Conversion2/1  "<IPM_Object_Length_17>"
  Bus Selector1/13 -> Data Type Conversion1/1  "<IPM_Object_Height_17>"
  Data Type Conversion17/1 -> Mux1/2
  Data Type Conversion18/1 -> Mux1/3
  Data Type Conversion16/1 -> Mux1/1
  Data Type Conversion24/1 -> Mux1/9
  Data Type Conversion22/1 -> Mux1/7
  Data Type Conversion20/1 -> Mux1/5
  Data Type Conversion19/1 -> Mux1/4
  Data Type Conversion25/1 -> Mux1/10
  Data Type Conversion23/1 -> Mux1/8
  Data Type Conversion21/1 -> Mux1/6
  Data Type Conversion26/1 -> Mux1/11
  Data Type Conversion27/1 -> Mux1/12
  Bus Selector1/1 -> Data Type Conversion16/1  "<IPM_ObjBlockCounter_17>"
  VR_ADCU_MRR_ObjHeader_0x680FromOutData/1 -> Bus Selector1/1
  Bus Selector1/2 -> Data Type Conversion17/1  "<IPM_ObjDistX_17>"
  Mux1/1 -> Out2/1
  Bus Selector1/3 -> Data Type Conversion18/1  "<IPM_ObjDistY_17>"
  Bus Selector1/6 -> Data Type Conversion21/1  "<IPM_ObjRelAccelY_17>"
  Bus Selector1/8 -> Data Type Conversion23/1  "<IPM_ObjRelVelY_17>"
  Bus Selector1/4 -> Data Type Conversion19/1  "<IPM_ObjID_17>"
  Bus Selector1/5 -> Data Type Conversion20/1  "<IPM_ObjRelAccelX_17>"
  Bus Selector1/7 -> Data Type Conversion22/1  "<IPM_ObjRelVelX_17>"
  Bus Selector1/9 -> Data Type Conversion24/1  "<IPM_ObjType_17>"
  Bus Selector1/11 -> Data Type Conversion26/1  "<IPM_Object_Existence_Probability_17>"
  Bus Selector1/10 -> Data Type Conversion25/1  "<IPM_Object_Age_17>"
  Bus Selector1/12 -> Data Type Conversion27/1  "<IPM_Object_Heading_17>"

== system ALL_JP360_DBW_V6_5_1103/MsgFromCAN/Subsystem1/Subsystem16 ==
  VR_ADCU_MRR_ObjHeader_0x680FromOutData : Inport
  Bus Selector1 : BusSelector  OutputSignals=IPM_ObjBlockCounter_10,IPM_ObjDistX_10,IPM_ObjDistY_10,IPM_ObjID_10,IPM_ObjRelAccelX_10,IPM_ObjRelAccelY_10,IPM_ObjRelVelX_10,IPM_ObjRelVelY_10,IPM_ObjType_10,IPM_Object_Age_10,IPM_Object_Existence_Probability_10,IPM_Object_Heading_10,IPM_Object_Height_10,IPM_Object_Length_10,IPM_Object_Motion_Status_10,IPM_Object_Width_10
  Data Type Conversion{1..2,4,6,16..27} (16 alike) : DataTypeConversion  OutDataTypeStr=single  SaturateOnIntegerOverflow=off  RndMeth=Floor
  Mux1 : Mux  Inputs=16
  Out2 : Outport
  wires:
  Bus Selector1/12 -> Data Type Conversion27/1  "<IPM_Object_Heading_10>"
  Bus Selector1/10 -> Data Type Conversion25/1  "<IPM_Object_Age_10>"
  Bus Selector1/11 -> Data Type Conversion26/1  "<IPM_Object_Existence_Probability_10>"
  Bus Selector1/9 -> Data Type Conversion24/1  "<IPM_ObjType_10>"
  Bus Selector1/7 -> Data Type Conversion22/1  "<IPM_ObjRelVelX_10>"
  Bus Selector1/5 -> Data Type Conversion20/1  "<IPM_ObjRelAccelX_10>"
  Bus Selector1/4 -> Data Type Conversion19/1  "<IPM_ObjID_10>"
  Bus Selector1/8 -> Data Type Conversion23/1  "<IPM_ObjRelVelY_10>"
  Bus Selector1/6 -> Data Type Conversion21/1  "<IPM_ObjRelAccelY_10>"
  Bus Selector1/3 -> Data Type Conversion18/1  "<IPM_ObjDistY_10>"
  Mux1/1 -> Out2/1
  Bus Selector1/2 -> Data Type Conversion17/1  "<IPM_ObjDistX_10>"
  VR_ADCU_MRR_ObjHeader_0x680FromOutData/1 -> Bus Selector1/1
  Bus Selector1/1 -> Data Type Conversion16/1  "<IPM_ObjBlockCounter_10>"
  Data Type Conversion27/1 -> Mux1/12
  Data Type Conversion26/1 -> Mux1/11
  Data Type Conversion21/1 -> Mux1/6
  Data Type Conversion23/1 -> Mux1/8
  Data Type Conversion25/1 -> Mux1/10
  Data Type Conversion19/1 -> Mux1/4
  Data Type Conversion20/1 -> Mux1/5
  Data Type Conversion22/1 -> Mux1/7
  Data Type Conversion24/1 -> Mux1/9
  Data Type Conversion16/1 -> Mux1/1
  Data Type Conversion18/1 -> Mux1/3
  Data Type Conversion17/1 -> Mux1/2
  Bus Selector1/13 -> Data Type Conversion1/1  "<IPM_Object_Height_10>"
  Bus Selector1/14 -> Data Type Conversion2/1  "<IPM_Object_Length_10>"
  Bus Selector1/15 -> Data Type Conversion4/1  "<IPM_Object_Motion_Status_10>"
  Bus Selector1/16 -> Data Type Conversion6/1  "<IPM_Object_Width_10>"
  Data Type Conversion1/1 -> Mux1/13
  Data Type Conversion2/1 -> Mux1/14
  Data Type Conversion4/1 -> Mux1/15
  Data Type Conversion6/1 -> Mux1/16
